simulink model "Telescope_model_PID"  (R2024b)
settings: Solver=ode4  StartTime=0.0  StopTime=SimulationTime  FixedStep=Tc  RelTol=1e-5
undefined symbols (not defined in the file): Arcs2Deg, Deg2Arcs, Kd_az, Kd_el, Ki_az, Ki_el, Kp_az, Kp_el, Kv, Prepocessor, Scenario, sgn, sysAz, sysEL, VonKarman
libraries: simulink x16
(part 1 of 2)
settings Model: Creator=giaco  LastModifiedBy=giacomobasile
settings RTWCC: GPUComputeCapability=3.5

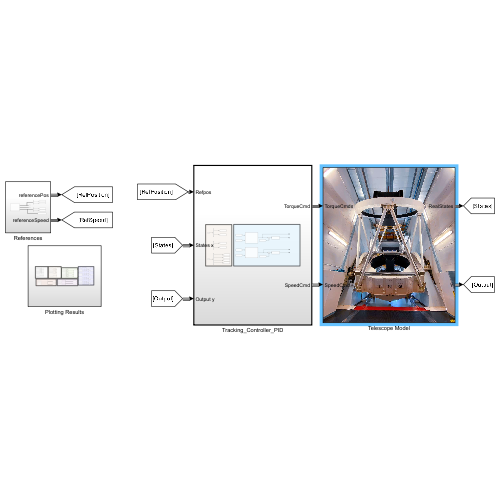
[thumbnail: Simulink's stored preview of the top-level diagram]
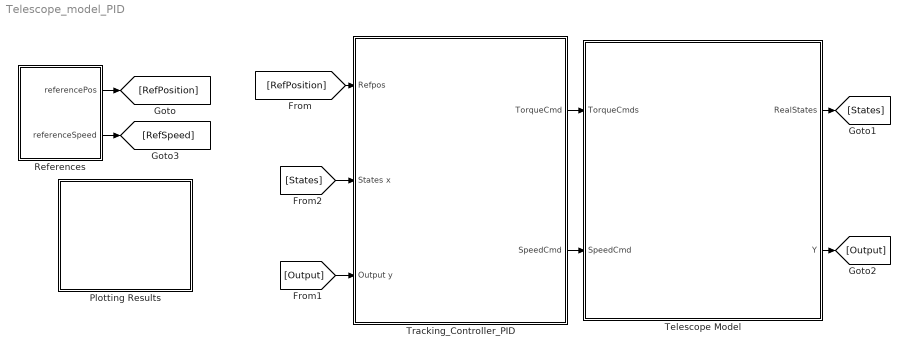
== system Telescope_model_PID ==
  Plotting Results : Subsystem
  References : Subsystem
  Telescope Model : Subsystem
      mask Display: image('tng1.jpg');
  Tracking_Controller_PID : Subsystem  TreatAsAtomicUnit=on  VariantControl=CtrMode == 1
  wires:
  Telescope Model/1(RealStates) -> [States]
  Telescope Model/2(Y) -> [Output]
  References/1(referencePos) -> [RefPosition]
  [RefPosition] -> Tracking_Controller_PID/1(Refpos)
  [States] -> Tracking_Controller_PID/2(States x)
  [Output] -> Tracking_Controller_PID/3(Output y)
  Tracking_Controller_PID/1(TorqueCmd) -> Telescope Model/1(TorqueCmds)
  Tracking_Controller_PID/2(SpeedCmd) -> Telescope Model/2(SpeedCmd)
  References/2(referenceSpeed) -> [RefSpeed]

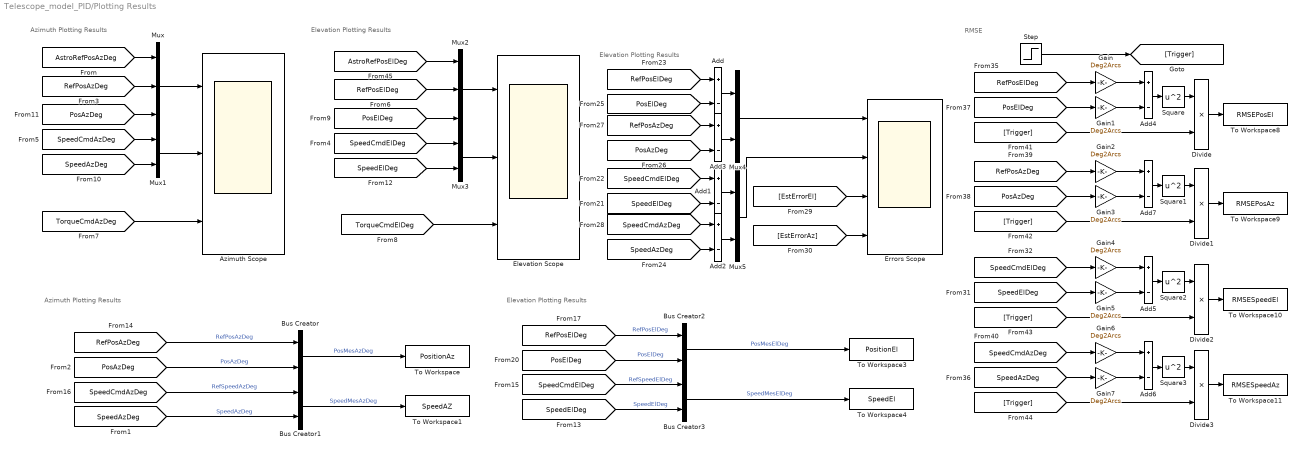
== system Telescope_model_PID/Plotting Results ==
  note: RMSE
  note: Azimuth Plotting Results
  note: Elevation Plotting Results
  note: Elevation Plotting Results
  note: Azimuth Plotting Results
  note: Elevation Plotting Results
  Add{,1..7} (8 alike) : Sum  Inputs=+-
  Azimuth Scope : Scope  NumInputPorts=3
  Bus Creator{,1..3} (4 alike) : BusCreator  Inputs=2
  Divide{,1..3} (4 alike) : Product  Inputs=**
  Elevation Scope : Scope  NumInputPorts=3
  Errors Scope : Scope  NumInputPorts=4
  Gain{,1..7} (8 alike) : Gain  Gain=Deg2Arcs
  Mux : Mux  Inputs=3
  Mux{1,3..5} (4 alike) : Mux  Inputs=2
  Mux2 : Mux  Inputs=3
  Square{,1..3} (4 alike) : Math  Operator=square
  Step : Step  Time=350  SampleTime=0
  To Workspace : ToWorkspace  VariableName=PositionAz  SaveFormat=Timeseries  SampleTime=-1
  To Workspace1 : ToWorkspace  VariableName=SpeedAZ  SaveFormat=Timeseries  SampleTime=-1
  To Workspace10 : ToWorkspace  VariableName=RMSESpeedEl  SaveFormat=Timeseries  SampleTime=-1
  To Workspace11 : ToWorkspace  VariableName=RMSESpeedAz  SaveFormat=Timeseries  SampleTime=-1
  To Workspace3 : ToWorkspace  VariableName=PositionEl  SaveFormat=Timeseries  SampleTime=-1
  To Workspace4 : ToWorkspace  VariableName=SpeedEl  SaveFormat=Timeseries  SampleTime=-1
  To Workspace8 : ToWorkspace  VariableName=RMSEPosEl  SaveFormat=Timeseries  SampleTime=-1
  To Workspace9 : ToWorkspace  VariableName=RMSEPosAz  SaveFormat=Timeseries  SampleTime=-1
  wires:
  [RefPosAzDeg] -> Mux/2
  [PosAzDeg] -> Mux/3
  [SpeedCmdAzDeg] -> Mux1/1
  [SpeedAzDeg] -> Mux1/2
  Mux/1 -> Azimuth Scope/1
  Mux1/1 -> Azimuth Scope/2
  [TorqueCmdAzDeg] -> Azimuth Scope/3
  [TorqueCmdElDeg] -> Elevation Scope/3
  Mux3/1 -> Elevation Scope/2
  Mux2/1 -> Elevation Scope/1
  [SpeedElDeg] -> Mux3/2
  [SpeedCmdElDeg] -> Mux3/1
  [PosElDeg] -> Mux2/3
  [RefPosElDeg] -> Mux2/2
  [PosAzDeg] -> Bus Creator/2  "PosAzDeg"
  [SpeedAzDeg] -> Bus Creator1/2  "SpeedAzDeg"
  [RefPosAzDeg] -> Bus Creator/1  "RefPosAzDeg"
  [SpeedCmdAzDeg] -> Bus Creator1/1  "RefSpeedAzDeg"
  [RefPosElDeg] -> Bus Creator2/1  "RefPosElDeg"
  [PosElDeg] -> Bus Creator2/2  "PosElDeg"
  [SpeedCmdElDeg] -> Bus Creator3/1  "RefSpeedElDeg"
  [SpeedElDeg] -> Bus Creator3/2  "SpeedElDeg"
  Bus Creator/1 -> To Workspace/1  "PosMesAzDeg"
  Bus Creator1/1 -> To Workspace1/1  "SpeedMesAzDeg"
  Bus Creator2/1 -> To Workspace3/1  "PosMesElDeg"
  Bus Creator3/1 -> To Workspace4/1  "SpeedMesElDeg"
  [RefPosElDeg] -> Add/1
  [PosElDeg] -> Add/2
  [SpeedCmdElDeg] -> Add1/1
  [SpeedElDeg] -> Add1/2
  [SpeedCmdAzDeg] -> Add2/1
  [SpeedAzDeg] -> Add2/2
  [RefPosAzDeg] -> Add3/1
  [PosAzDeg] -> Add3/2
  Add/1 -> Mux4/1
  Add3/1 -> Mux4/2
  Add1/1 -> Mux5/1
  Add2/1 -> Mux5/2
  Mux4/1 -> Errors Scope/1
  Mux5/1 -> Errors Scope/2
  [EstErrorEl] -> Errors Scope/3
  [EstErrorAz] -> Errors Scope/4
  Add6/1 -> Square3/1
  Add5/1 -> Square2/1
  Add7/1 -> Square1/1
  Add4/1 -> Square/1
  [PosAzDeg] -> Gain3/1
  [RefPosAzDeg] -> Gain2/1
  [SpeedAzDeg] -> Gain7/1
  [SpeedCmdAzDeg] -> Gain6/1
  [SpeedElDeg] -> Gain5/1
  [SpeedCmdElDeg] -> Gain4/1
  [PosElDeg] -> Gain1/1
  [RefPosElDeg] -> Gain/1
  Square/1 -> Divide/1
  Divide/1 -> To Workspace8/1
  Step/1 -> [Trigger]
  [Trigger] -> Divide/2
  [Trigger] -> Divide1/2
  Square1/1 -> Divide1/1
  Divide1/1 -> To Workspace9/1
  [Trigger] -> Divide2/2
  Square2/1 -> Divide2/1
  Divide2/1 -> To Workspace10/1
  [Trigger] -> Divide3/2
  Square3/1 -> Divide3/1
  Divide3/1 -> To Workspace11/1
  Gain/1 -> Add4/1
  Gain1/1 -> Add4/2
  Gain2/1 -> Add7/1
  Gain3/1 -> Add7/2
  Gain4/1 -> Add5/1
  Gain5/1 -> Add5/2
  Gain6/1 -> Add6/1
  Gain7/1 -> Add6/2
  [AstroRefPosElDeg] -> Mux2/1
  [AstroRefPosAzDeg] -> Mux/1

== system Telescope_model_PID/References ==
  Bus Selector : BusSelector  OutputSignals=Azimuth,Elevation
  Bus Selector1 : BusSelector  OutputSignals=ElevationPosition,AzimuthPosition
  References : Subsystem  Variant=on  VariantControl=Choice
  To Workspace : ToWorkspace  VariableName=AstroReference  SaveFormat=Timeseries  SampleTime=-1
  referencePos : Outport
  referenceSpeed : Outport  Port=2
  tag scope: AstroRefPosAzDeg=global, AstroRefPosElDeg=global, RefPosAzDeg=global, RefPosElDeg=global
  wires:
  References/1(referencePos) -> Bus Selector/1, referencePos/1  "[Arcs]"
  Bus Selector/1 -> [RefPosAzDeg]  "<Azimuth>"
  Bus Selector/2 -> [RefPosElDeg]  "<Elevation>"
  References/2(referenceSpeed) -> referenceSpeed/1  "[Arcs]"
  Bus Selector1/2 -> [AstroRefPosAzDeg]  "<AzimuthPosition>"
  Bus Selector1/1 -> [AstroRefPosElDeg]  "<ElevationPosition>"
  References/3(AstroReference) -> To Workspace/1, Bus Selector1/1  "[Arcs]"

== system Telescope_model_PID/Telescope Model ==
  note: Input Management Section
  note: Models dynamics
  TorqueCmds : Inport
  SpeedCmd : Inport  Port=2
  Azimuth Model 50 deg : Subsystem
  Bus Selector : BusSelector  OutputSignals=Elevation,Azimuth50
  Bus Selector1 : BusSelector  OutputSignals=Elevation,Azimuth50
  Elevation Model : Subsystem
  Integrator : Integrator  InitialCondition=Prepocessor.p0el*Deg2Arcs
  Integrator1 : Integrator  InitialCondition=Prepocessor.p0az*Deg2Arcs
  To Workspace1 : ToWorkspace  VariableName=TorqueAz  SaveFormat=Timeseries  SampleTime=-1
  To Workspace3 : ToWorkspace  VariableName=TorqueEl  SaveFormat=Timeseries  SampleTime=-1
  Transfer Fcn1 : TransferFcn  Numerator=10000  Denominator=conv([1 100], [1 100])
  Transfer Fcn2 : TransferFcn  Numerator=10000  Denominator=conv([1 100], [1 100])
  Out Bus Element : Outport  PortName=RealStates  Element=Elevation
  Out Bus Element1 : Outport  PortName=RealStates  Element=Azimuth50
  Out Bus Element2 : Outport  Port=2  PortName=Y  Element=ElevationSpeed
  Out Bus Element3 : Outport  Port=2  PortName=Y  Element=ElevationPosition
  Out Bus Element4 : Outport  Port=2  PortName=Y  Element=Azimuth50Speed
  Out Bus Element5 : Outport  Port=2  PortName=Y  Element=Azimuth50Position
  tag scope: PosAzDeg=global, PosElDeg=global, SpeedAzDeg=global, SpeedCmdAzDeg=global, SpeedCmdElDeg=global, SpeedElDeg=global, TorqueCmdAzDeg=global, TorqueCmdElDeg=global
  wires:
  Elevation Model/1(x) -> Out Bus Element/1
  Azimuth Model 50 deg/1(x) -> Out Bus Element1/1
  TorqueCmds/1 -> Bus Selector/1
  Azimuth Model 50 deg/2(y) -> [SpeedAzDeg], Out Bus Element4/1, Integrator1/1
  Elevation Model/2(y) -> [SpeedElDeg], Out Bus Element2/1, Integrator/1
  Integrator1/1 -> [PosAzDeg], Out Bus Element5/1
  Integrator/1 -> [PosElDeg], Out Bus Element3/1
  Bus Selector1/2 -> Transfer Fcn1/1  "<Azimuth50>"
  Bus Selector/1 -> To Workspace3/1, [TorqueCmdElDeg]  "<Elevation>"
  Bus Selector1/1 -> Transfer Fcn2/1  "<Elevation>"
  Bus Selector/2 -> To Workspace1/1, [TorqueCmdAzDeg]  "<Azimuth50>"
  [TorqueCmdElDeg] -> Elevation Model/1(Torque)
  [TorqueCmdAzDeg] -> Azimuth Model 50 deg/1(Troque)
  SpeedCmd/1 -> Bus Selector1/1
  Transfer Fcn2/1 -> [SpeedCmdElDeg]
  Transfer Fcn1/1 -> [SpeedCmdAzDeg]

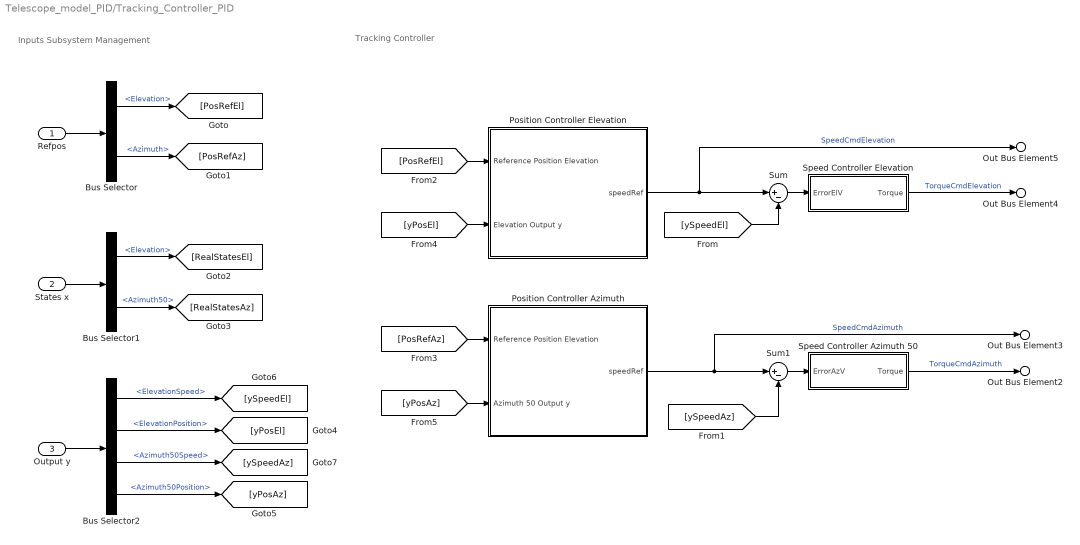
== system Telescope_model_PID/Tracking_Controller_PID ==
  note: Inputs Subsystem Management
  note: Tracking Controller
  Refpos : Inport
  States x : Inport  Port=2
  Output y : Inport  Port=3
  Bus Selector : BusSelector  OutputSignals=Elevation,Azimuth
  Bus Selector1 : BusSelector  OutputSignals=Elevation,Azimuth50
  Bus Selector2 : BusSelector  OutputSignals=ElevationSpeed,ElevationPosition,Azimuth50Speed,Azimuth50Position
  Position Controller Azimuth : Subsystem
  Position Controller Elevation : Subsystem
  Speed Controller Azimuth 50 : Subsystem
  Speed Controller Elevation : Subsystem
  Sum : Sum  Inputs=|+-
  Sum1 : Sum  Inputs=|+-
  Out Bus Element2 : Outport  PortName=TorqueCmd  Element=Azimuth50
  Out Bus Element4 : Outport  PortName=TorqueCmd  Element=Elevation
  Out Bus Element3 : Outport  Port=2  PortName=SpeedCmd  Element=Azimuth50
  Out Bus Element5 : Outport  Port=2  PortName=SpeedCmd  Element=Elevation
  wires:
  Position Controller Azimuth/1(speedRef) -> Sum1/1, Out Bus Element3/1  "SpeedCmdAzimuth"
  [PosRefEl] -> Position Controller Elevation/1(Reference Position Elevation)
  Sum/1 -> Speed Controller Elevation/1(ErrorElV)
  Sum1/1 -> Speed Controller Azimuth 50/1(ErrorAzV)
  [ySpeedAz] -> Sum1/2
  Speed Controller Azimuth 50/1(Torque) -> Out Bus Element2/1  "TorqueCmdAzimuth"
  Speed Controller Elevation/1(Torque) -> Out Bus Element4/1  "TorqueCmdElevation"
  Position Controller Elevation/1(speedRef) -> Sum/1, Out Bus Element5/1  "SpeedCmdElevation"
  [PosRefAz] -> Position Controller Azimuth/1(Reference Position Elevation)
  [ySpeedEl] -> Sum/2
  Bus Selector2/2 -> [yPosEl]  "<ElevationPosition>"
  Bus Selector2/1 -> [ySpeedEl]  "<ElevationSpeed>"
  Bus Selector2/3 -> [ySpeedAz]  "<Azimuth50Speed>"
  Bus Selector2/4 -> [yPosAz]  "<Azimuth50Position>"
  Output y/1 -> Bus Selector2/1
  Bus Selector1/2 -> [RealStatesAz]  "<Azimuth50>"
  Bus Selector1/1 -> [RealStatesEl]  "<Elevation>"
  States x/1 -> Bus Selector1/1
  Bus Selector/2 -> [PosRefAz]  "<Azimuth>"
  Bus Selector/1 -> [PosRefEl]  "<Elevation>"
  Refpos/1 -> Bus Selector/1
  [yPosEl] -> Position Controller Elevation/2(Elevation Output y)
  [yPosAz] -> Position Controller Azimuth/2(Azimuth 50 Output y)

== system Telescope_model_PID/References/References ==
  Astrometric Computation : Subsystem  VariantControl=Ref == 0 && Prepocessor.flag == 0 && TNG==0
  Constant Referemce : Subsystem  VariantControl=Ref == 2
  Preprocessed Astrometric Computation : Subsystem  VariantControl=Ref == 0 && Prepocessor.flag == 1 && TNG==0
  Preprocessed Astrometric References from TNG : Subsystem  VariantControl=Ref == 0 && Prepocessor.flag == 1 && TNG==1
  Trivial References PID/LQG : Subsystem  VariantControl=Ref == 1
  referencePos : Outport
  referenceSpeed : Outport  Port=2
  AstroReference : Outport  Port=3

== system Telescope_model_PID/Telescope Model/Azimuth Model 50 deg ==
  Troque : Inport
  Add : Sum
  Add1 : Sum
  Integrator : Integrator
  Noise Model : Subsystem  Variant=on  VariantControl=Choice
  Scope : Scope  NumInputPorts=2
  Sum : Sum  Inputs=++|
  Sum1 : Sum  Inputs=++|
  sys.A : Gain  Gain=sysAz.A  Multiplication=Matrix(K*u)
  sys.B : Gain  Gain=sysAz.B  Multiplication=Matrix(K*u)
  sys.C : Gain  Gain=sysAz.C  Multiplication=Matrix(K*u)
  sys.D : Gain  Gain=sysAz.D  Multiplication=Matrix(K*u)
  x : Outport
  y : Outport  Port=2
  tag scope: InputNoiseAz=global
  wires:
  Add1/1 -> Integrator/1
  sys.C/1 -> Add/2
  sys.D/1 -> Add/1
  Sum1/1 -> sys.B/1, sys.D/1
  Sum/1 -> y/1
  Add/1 -> Sum/2
  Troque/1 -> Sum1/2
  Noise Model/1(d_out) -> Scope/1, Sum/1
  sys.B/1 -> Add1/1
  sys.A/1 -> Add1/2
  Integrator/1 -> sys.A/1, sys.C/1, x/1
  Noise Model/2(d_in) -> [InputNoiseAz], Sum1/1, Scope/2

== system Telescope_model_PID/Telescope Model/Elevation Model ==
  Torque : Inport
  Add : Sum
  Add1 : Sum
  Integrator : Integrator
  Noise Model : Subsystem  Variant=on  VariantControl=Choice
  Scope : Scope  NumInputPorts=2
  Sum : Sum  Inputs=++|
  Sum1 : Sum  Inputs=++|
  sys.A : Gain  Gain=sysEL.A  Multiplication=Matrix(K*u)
  sys.B : Gain  Gain=sysEL.B  Multiplication=Matrix(K*u)
  sys.C : Gain  Gain=sysEL.C  Multiplication=Matrix(K*u)
  sys.D : Gain  Gain=sysEL.D  Multiplication=Matrix(K*u)
  x : Outport
  y : Outport  Port=2
  tag scope: InputNoiseEl=global
  wires:
  sys.B/1 -> Add1/1
  sys.C/1 -> Add/2
  sys.D/1 -> Add/1
  Add/1 -> Sum/2
  Sum/1 -> y/1
  Sum1/1 -> sys.B/1, sys.D/1
  Torque/1 -> Sum1/2
  Noise Model/1(d_out) -> Scope/1, Sum/1
  Noise Model/2(d_in) -> [InputNoiseEl], Sum1/1, Scope/2
  sys.A/1 -> Add1/2
  Add1/1 -> Integrator/1
  Integrator/1 -> sys.A/1, x/1, sys.C/1

== system Telescope_model_PID/Tracking_Controller_PID/Position Controller Azimuth ==
  note: Inputs Subsystem Management
  note: Controller PID
  Reference Position Elevation : Inport
  Azimuth 50 Output y : Inport  Port=2
  Add4 : Sum  Inputs=+++
  Gain1 : Gain  Gain=Kd_az  Multiplication=Matrix(K*u)
  Gain5 : Gain  Gain=Kp_az  Multiplication=Matrix(K*u)
  Gain6 : Gain  Gain=Ki_az  Multiplication=Matrix(K*u)
  Integrator : Integrator
  Sum : Sum  Inputs=+-|
  Transfer Fcn : TransferFcn  Numerator=[100 0]  Denominator=[1 100]
  speedRef : Outport
  wires:
  Reference Position Elevation/1 -> Sum/1
  Azimuth 50 Output y/1 -> Sum/2
  Sum/1 -> [ErrorP]
  Add4/1 -> speedRef/1
  Transfer Fcn/1 -> Gain1/1
  [ErrorP] -> Gain5/1, Transfer Fcn/1, Integrator/1
  Gain6/1 -> Add4/2
  Gain5/1 -> Add4/1
  Integrator/1 -> Gain6/1
  Gain1/1 -> Add4/3

== system Telescope_model_PID/Tracking_Controller_PID/Position Controller Elevation ==
  note: Inputs Subsystem Management
  note: Controller PID
  Reference Position Elevation : Inport
  Elevation Output y : Inport  Port=2
  Add4 : Sum  Inputs=+++
  Gain1 : Gain  Gain=Kd_el  Multiplication=Matrix(K*u)
  Gain5 : Gain  Gain=Kp_el  Multiplication=Matrix(K*u)
  Gain6 : Gain  Gain=Ki_el  Multiplication=Matrix(K*u)
  Integrator : Integrator
  Sum : Sum  Inputs=+-|
  Transfer Fcn : TransferFcn  Numerator=[100 0]  Denominator=[1 100]
  speedRef : Outport
  wires:
  Reference Position Elevation/1 -> Sum/1
  Gain6/1 -> Add4/2
  Integrator/1 -> Gain6/1
  [ErrorP] -> Gain5/1, Transfer Fcn/1, Integrator/1
  Gain5/1 -> Add4/1
  Sum/1 -> [ErrorP]
  Elevation Output y/1 -> Sum/2
  Add4/1 -> speedRef/1
  Transfer Fcn/1 -> Gain1/1
  Gain1/1 -> Add4/3

== system Telescope_model_PID/Tracking_Controller_PID/Speed Controller Azimuth 50 ==
  ErrorAzV : Inport
  Gain : Gain  Gain=Kv
  Integrator : Integrator
  Torque : Outport
  wires:
  Gain/1 -> Torque/1
  ErrorAzV/1 -> Integrator/1
  Integrator/1 -> Gain/1

== system Telescope_model_PID/Tracking_Controller_PID/Speed Controller Elevation ==
  ErrorElV : Inport
  Gain : Gain  Gain=-Kv
  Integrator : Integrator
  Torque : Outport
  wires:
  Integrator/1 -> Gain/1
  ErrorElV/1 -> Integrator/1
  Gain/1 -> Torque/1

== system Telescope_model_PID/References/References/Astrometric Computation ==
  Clock : Clock
  Constant10 : Constant  Value=Scenario.VLT
  Constant11 : Constant  Value=Scenario.Time
  Constant19 : Constant  Value=Scenario.RAhh
  Constant21 : Constant  Value=Scenario.DECdd
  Constant3 : Constant  Value=Scenario.RAmm
  Constant4 : Constant  Value=Scenario.RAss
  Constant6 : Constant  Value=Scenario.DECmm
  Constant7 : Constant  Value=Scenario.DECss
  Constant8 : Constant  Value=Scenario.LATsite
  Constant9 : Constant  Value=Scenario.LONsite
  Discrete Derivative{,1..3} (4 alike) : simulink/Discrete/Discrete Derivative  gainval=1.0  ICPrevScaledInput=0.0  OutMin=[]  OutMax=[]  OutDataType=fixdt(1, 16)  OutScaling=2^-10  DoSatur=off
  MATLAB Function : MATLAB Function  TreatAsAtomicUnit=on
  Scope2 : Scope
  Out Bus Element : Outport  PortName=referencePos  Element=Azimuth
  Out Bus Element1 : Outport  PortName=referencePos  Element=Elevation
  Out Bus Element2 : Outport  Port=2  PortName=referenceSpeed  Element=Azimuth
  Out Bus Element3 : Outport  Port=2  PortName=referenceSpeed  Element=Elevation
  Out Bus Element4 : Outport  Port=3  PortName=AstroReference  Element=AzimuthSpeed
  Out Bus Element5 : Outport  Port=3  PortName=AstroReference  Element=ElevationPosition
  Out Bus Element6 : Outport  Port=3  PortName=AstroReference  Element=AzimuthPosition
  Out Bus Element7 : Outport  Port=3  PortName=AstroReference  Element=ElevationSpeed
  wires:
  Discrete Derivative1/1 -> Out Bus Element7/1
  Constant9/1 -> MATLAB Function/10(Longitude)
  Constant19/1 -> MATLAB Function/3(RAhh)
  Constant3/1 -> MATLAB Function/4(RAmm)
  Constant21/1 -> MATLAB Function/6(DECdd)
  Clock/1 -> Scope2/1, MATLAB Function/1(clo)
  Discrete Derivative3/1 -> Out Bus Element3/1
  Constant4/1 -> MATLAB Function/5(RAss)
  Constant7/1 -> MATLAB Function/8(DECss)
  Constant6/1 -> MATLAB Function/7(DECmm)
  Constant10/1 -> MATLAB Function/11(VLT)
  Constant11/1 -> MATLAB Function/2(Time)
  Discrete Derivative2/1 -> Out Bus Element2/1
  Constant8/1 -> MATLAB Function/9(Latitude)
  MATLAB Function/1(Az) -> Discrete Derivative/1, Out Bus Element6/1, Discrete Derivative2/1, Out Bus Element/1
  MATLAB Function/2(Alt) -> Discrete Derivative3/1, Out Bus Element5/1, Discrete Derivative1/1, Out Bus Element1/1
  Discrete Derivative/1 -> Out Bus Element4/1

== system Telescope_model_PID/References/References/Constant Referemce ==
  Constant2 : Constant  Value=0
  Constant3 : Constant  Value=0
  Discrete Derivative : simulink/Discrete/Discrete Derivative  gainval=1.0  ICPrevScaledInput=0.0  OutMin=[]  OutMax=[]  OutDataType=fixdt(1, 16)  OutScaling=2^-10  DoSatur=off
  Discrete Derivative1 : simulink/Discrete/Discrete Derivative  gainval=1.0  ICPrevScaledInput=0.0  OutMin=[]  OutMax=[]  OutDataType=fixdt(1, 16)  OutScaling=2^-10  DoSatur=off
  Gain{6..13} (8 alike) : Gain  Gain=Deg2Arcs
  Integrator3 : Integrator  InitialCondition=120
  Integrator4 : Integrator  InitialCondition=60
  Prepocessor Azimuth : Subsystem
  Prepocessor Elavation : Subsystem
  Out Bus Element : Outport  PortName=referencePos  Element=Azimuth
  Out Bus Element1 : Outport  PortName=referencePos  Element=Elevation
  Out Bus Element2 : Outport  Port=2  PortName=referenceSpeed  Element=Azimuth
  Out Bus Element3 : Outport  Port=2  PortName=referenceSpeed  Element=Elevation
  Out Bus Element4 : Outport  Port=3  PortName=AstroReference  Element=AzimuthSpeed
  Out Bus Element5 : Outport  Port=3  PortName=AstroReference  Element=ElevationPosition
  Out Bus Element6 : Outport  Port=3  PortName=AstroReference  Element=AzimuthPosition
  Out Bus Element7 : Outport  Port=3  PortName=AstroReference  Element=ElevationSpeed
  wires:
  Integrator3/1 -> Discrete Derivative1/1, Gain8/1, Prepocessor Azimuth/1(Astrometry Computation)  "[Deg]"
  Integrator4/1 -> Prepocessor Elavation/1(Astrometry Computation), Discrete Derivative/1, Gain11/1  "[Deg]"
  Prepocessor Elavation/1(ReferencePosition) -> Gain12/1
  Prepocessor Azimuth/1(ReferencePosition) -> Gain6/1
  Gain8/1 -> Out Bus Element6/1
  Gain10/1 -> Out Bus Element7/1
  Gain11/1 -> Out Bus Element5/1
  Gain6/1 -> Out Bus Element/1
  Gain13/1 -> Out Bus Element3/1
  Gain7/1 -> Out Bus Element2/1
  Discrete Derivative1/1 -> Gain9/1
  Discrete Derivative/1 -> Gain10/1
  Gain12/1 -> Out Bus Element1/1
  Prepocessor Elavation/2(ReferenceSpeed) -> Gain13/1
  Constant3/1 -> Integrator4/1  "[Deg]"
  Gain9/1 -> Out Bus Element4/1
  Constant2/1 -> Integrator3/1  "[Deg]"
  Prepocessor Azimuth/2(ReferenceSpeed) -> Gain7/1

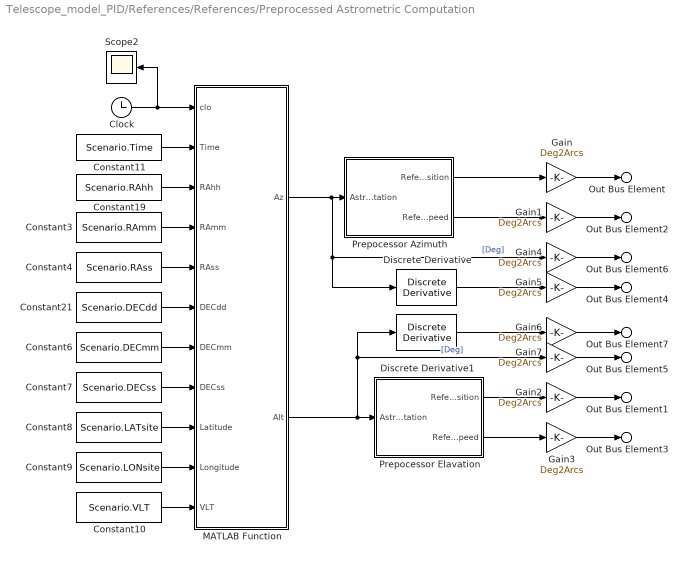
== system Telescope_model_PID/References/References/Preprocessed Astrometric Computation ==
  Clock : Clock
  Constant10 : Constant  Value=Scenario.VLT
  Constant11 : Constant  Value=Scenario.Time
  Constant19 : Constant  Value=Scenario.RAhh
  Constant21 : Constant  Value=Scenario.DECdd
  Constant3 : Constant  Value=Scenario.RAmm
  Constant4 : Constant  Value=Scenario.RAss
  Constant6 : Constant  Value=Scenario.DECmm
  Constant7 : Constant  Value=Scenario.DECss
  Constant8 : Constant  Value=Scenario.LATsite
  Constant9 : Constant  Value=Scenario.LONsite
  Discrete Derivative : simulink/Discrete/Discrete Derivative  gainval=1.0  ICPrevScaledInput=0.0  OutMin=[]  OutMax=[]  OutDataType=fixdt(1, 16)  OutScaling=2^-10  DoSatur=off
  Discrete Derivative1 : simulink/Discrete/Discrete Derivative  gainval=1.0  ICPrevScaledInput=0.0  OutMin=[]  OutMax=[]  OutDataType=fixdt(1, 16)  OutScaling=2^-10  DoSatur=off
  Gain{,1..7} (8 alike) : Gain  Gain=Deg2Arcs
  MATLAB Function : MATLAB Function  TreatAsAtomicUnit=on
  Prepocessor Azimuth : Subsystem
  Prepocessor Elavation : Subsystem
  Scope2 : Scope
  Out Bus Element : Outport  PortName=referencePos  Element=Azimuth
  Out Bus Element1 : Outport  PortName=referencePos  Element=Elevation
  Out Bus Element2 : Outport  Port=2  PortName=referenceSpeed  Element=Azimuth
  Out Bus Element3 : Outport  Port=2  PortName=referenceSpeed  Element=Elevation
  Out Bus Element4 : Outport  Port=3  PortName=AstroReference  Element=AzimuthSpeed
  Out Bus Element5 : Outport  Port=3  PortName=AstroReference  Element=ElevationPosition
  Out Bus Element6 : Outport  Port=3  PortName=AstroReference  Element=AzimuthPosition
  Out Bus Element7 : Outport  Port=3  PortName=AstroReference  Element=ElevationSpeed
  wires:
  Constant21/1 -> MATLAB Function/6(DECdd)
  Constant7/1 -> MATLAB Function/8(DECss)
  Constant11/1 -> MATLAB Function/2(Time)
  Constant6/1 -> MATLAB Function/7(DECmm)
  Constant10/1 -> MATLAB Function/11(VLT)
  Clock/1 -> Scope2/1, MATLAB Function/1(clo)
  Constant4/1 -> MATLAB Function/5(RAss)
  Constant8/1 -> MATLAB Function/9(Latitude)
  Constant3/1 -> MATLAB Function/4(RAmm)
  Constant9/1 -> MATLAB Function/10(Longitude)
  Constant19/1 -> MATLAB Function/3(RAhh)
  MATLAB Function/1(Az) -> Gain4/1, Discrete Derivative/1, Prepocessor Azimuth/1(Astrometry Computation)  "[Deg]"
  MATLAB Function/2(Alt) -> Discrete Derivative1/1, Gain7/1, Prepocessor Elavation/1(Astrometry Computation)  "[Deg]"
  Prepocessor Azimuth/2(ReferenceSpeed) -> Gain1/1
  Prepocessor Azimuth/1(ReferencePosition) -> Gain/1
  Prepocessor Elavation/2(ReferenceSpeed) -> Gain3/1
  Prepocessor Elavation/1(ReferencePosition) -> Gain2/1
  Discrete Derivative/1 -> Gain5/1
  Discrete Derivative1/1 -> Gain6/1
  Gain/1 -> Out Bus Element/1
  Gain1/1 -> Out Bus Element2/1
  Gain2/1 -> Out Bus Element1/1
  Gain3/1 -> Out Bus Element3/1
  Gain4/1 -> Out Bus Element6/1
  Gain5/1 -> Out Bus Element4/1
  Gain6/1 -> Out Bus Element7/1
  Gain7/1 -> Out Bus Element5/1

== system Telescope_model_PID/References/References/Preprocessed Astrometric References from TNG ==
  Discrete Derivative : simulink/Discrete/Discrete Derivative  gainval=1.0  ICPrevScaledInput=0.0  OutMin=[]  OutMax=[]  OutDataType=fixdt(1, 16)  OutScaling=2^-10  DoSatur=off
  Discrete Derivative1 : simulink/Discrete/Discrete Derivative  gainval=1.0  ICPrevScaledInput=0.0  OutMin=[]  OutMax=[]  OutDataType=fixdt(1, 16)  OutScaling=2^-10  DoSatur=off
  From Workspace : FromWorkspace  VariableName=Scenario.AzimuthPosition
  From Workspace1 : FromWorkspace  VariableName=Scenario.ElevationPosition
  Gain : Gain  Gain=Arcs2Deg
  Gain1 : Gain  Gain=Arcs2Deg
  Gain{2..9} (8 alike) : Gain  Gain=Deg2Arcs
  Prepocessor Azimuth : Subsystem
  Prepocessor Elavation : Subsystem
  Out Bus Element : Outport  PortName=referencePos  Element=Azimuth
  Out Bus Element1 : Outport  PortName=referencePos  Element=Elevation
  Out Bus Element2 : Outport  Port=2  PortName=referenceSpeed  Element=Azimuth
  Out Bus Element3 : Outport  Port=2  PortName=referenceSpeed  Element=Elevation
  Out Bus Element4 : Outport  Port=3  PortName=AstroReference  Element=AzimuthSpeed
  Out Bus Element5 : Outport  Port=3  PortName=AstroReference  Element=ElevationPosition
  Out Bus Element6 : Outport  Port=3  PortName=AstroReference  Element=AzimuthPosition
  Out Bus Element7 : Outport  Port=3  PortName=AstroReference  Element=ElevationSpeed
  wires:
  Discrete Derivative/1 -> Gain6/1
  Discrete Derivative1/1 -> Gain5/1
  Prepocessor Elavation/1(ReferencePosition) -> Gain8/1
  Prepocessor Elavation/2(ReferenceSpeed) -> Gain9/1
  Prepocessor Azimuth/1(ReferencePosition) -> Gain2/1
  Prepocessor Azimuth/2(ReferenceSpeed) -> Gain3/1
  From Workspace/1 -> Gain/1  "[Arcs]"
  Gain/1 -> Prepocessor Azimuth/1(Astrometry Computation), Discrete Derivative1/1, Gain4/1  "[Deg]"
  Gain1/1 -> Prepocessor Elavation/1(Astrometry Computation), Discrete Derivative/1, Gain7/1  "[Deg]"
  From Workspace1/1 -> Gain1/1  "[Arcs]"
  Gain2/1 -> Out Bus Element/1
  Gain3/1 -> Out Bus Element2/1
  Gain4/1 -> Out Bus Element6/1
  Gain5/1 -> Out Bus Element4/1
  Gain6/1 -> Out Bus Element7/1
  Gain7/1 -> Out Bus Element5/1
  Gain8/1 -> Out Bus Element1/1
  Gain9/1 -> Out Bus Element3/1

== system Telescope_model_PID/References/References/Trivial References PID//LQG ==
  Add1 : Sum  Inputs=+-
  Add2 : Sum  Inputs=+-
  Discrete Derivative : simulink/Discrete/Discrete Derivative  gainval=1.0  ICPrevScaledInput=0.0  OutMin=[]  OutMax=[]  OutDataType=fixdt(1, 16)  OutScaling=2^-10  DoSatur=off
  Discrete Derivative1 : simulink/Discrete/Discrete Derivative  gainval=1.0  ICPrevScaledInput=0.0  OutMin=[]  OutMax=[]  OutDataType=fixdt(1, 16)  OutScaling=2^-10  DoSatur=off
  Gain{6..13} (8 alike) : Gain  Gain=Deg2Arcs
  Integrator1 : Integrator
  Integrator2 : Integrator
  Prepocessor Azimuth : Subsystem
  Prepocessor Elavation : Subsystem
  Step1 : Step  Time=2  After=5  SampleTime=0
  Step2 : Step  Time=12  After=5  SampleTime=0
  Step4 : Step  Time=20  After=0.2  SampleTime=0
  Step5 : Step  Time=30  After=0.2  SampleTime=0
  Out Bus Element : Outport  PortName=referencePos  Element=Azimuth
  Out Bus Element1 : Outport  PortName=referencePos  Element=Elevation
  Out Bus Element2 : Outport  Port=2  PortName=referenceSpeed  Element=Azimuth
  Out Bus Element3 : Outport  Port=2  PortName=referenceSpeed  Element=Elevation
  Out Bus Element4 : Outport  Port=3  PortName=AstroReference  Element=AzimuthSpeed
  Out Bus Element5 : Outport  Port=3  PortName=AstroReference  Element=ElevationPosition
  Out Bus Element6 : Outport  Port=3  PortName=AstroReference  Element=AzimuthPosition
  Out Bus Element7 : Outport  Port=3  PortName=AstroReference  Element=ElevationSpeed
  wires:
  Step4/1 -> Add2/1
  Step5/1 -> Add2/2
  Step2/1 -> Add1/2
  Step1/1 -> Add1/1
  Add1/1 -> Integrator1/1  "[Deg]"
  Add2/1 -> Integrator2/1  "[Deg]"
  Gain6/1 -> Out Bus Element/1
  Gain11/1 -> Out Bus Element5/1
  Gain10/1 -> Out Bus Element7/1
  Gain7/1 -> Out Bus Element2/1
  Gain13/1 -> Out Bus Element3/1
  Gain9/1 -> Out Bus Element4/1
  Prepocessor Azimuth/2(ReferenceSpeed) -> Gain7/1
  Prepocessor Azimuth/1(ReferencePosition) -> Gain6/1
  Prepocessor Elavation/1(ReferencePosition) -> Gain12/1
  Prepocessor Elavation/2(ReferenceSpeed) -> Gain13/1
  Gain8/1 -> Out Bus Element6/1
  Integrator1/1 -> Discrete Derivative1/1, Gain8/1, Prepocessor Azimuth/1(Astrometry Computation)  "[Deg]"
  Integrator2/1 -> Prepocessor Elavation/1(Astrometry Computation), Discrete Derivative/1, Gain11/1  "[Deg]"
  Gain12/1 -> Out Bus Element1/1
  Discrete Derivative1/1 -> Gain9/1
  Discrete Derivative/1 -> Gain10/1

== system Telescope_model_PID/Telescope Model/Azimuth Model 50 deg/Noise Model ==
  None Noise : Subsystem  VariantControl="NNFConf  == 0"
  Von Karman Torque PSD : Subsystem  VariantControl=NNFConf == 2
  White Noise Output : Subsystem  VariantControl=NNFConf == 1
  d_out : Outport
  d_in : Outport  Port=2

== system Telescope_model_PID/Telescope Model/Elevation Model/Noise Model ==
  None Noise : Subsystem  VariantControl="NNFConf  == 0"
  Von Karman Torque PSD : Subsystem  VariantControl=NNFConf == 2
  White Noise Output : Subsystem  VariantControl=NNFConf == 1
  d_out : Outport
  d_in : Outport  Port=2

== system Telescope_model_PID/References/References/Constant Referemce/Prepocessor Azimuth ==
  Astrometry Computation : Inport
  Integrator : Integrator  InitialCondition=Prepocessor.p0az
  Prepocessor Elevation : Subsystem  TreatAsAtomicUnit=on  SystemSampleTime=Prepocessor.Ts
  Terminator : Terminator
  Terminator1 : Terminator
  To Workspace : ToWorkspace  VariableName=ReferenceProcessedPositionAz  SaveFormat=Timeseries  SampleTime=-1
  To Workspace1 : ToWorkspace  VariableName=ReferenceProcessedSpeedAz  SaveFormat=Timeseries  SampleTime=-1
  Transfer Fcn2 : TransferFcn  Numerator=2500  Denominator=conv([1 50], [1 50])
  ReferencePosition : Outport
  ReferenceSpeed : Outport  Port=2
  wires:
  Prepocessor Elevation/2(speed) -> Transfer Fcn2/1
  Prepocessor Elevation/1(deltaP) -> Terminator/1
  Integrator/1 -> To Workspace/1, ReferencePosition/1
  Prepocessor Elevation/3(PositionRef) -> Terminator1/1
  Transfer Fcn2/1 -> To Workspace1/1, ReferenceSpeed/1, Integrator/1
  Astrometry Computation/1 -> Prepocessor Elevation/1(Az)

== system Telescope_model_PID/References/References/Constant Referemce/Prepocessor Elavation ==
  Astrometry Computation : Inport
  Integrator : Integrator  InitialCondition=Prepocessor.p0el
  Prepocessor Elevation : Subsystem  TreatAsAtomicUnit=on  SystemSampleTime=Prepocessor.Ts
  Terminator : Terminator
  Terminator1 : Terminator
  To Workspace : ToWorkspace  VariableName=ReferenceProcessedPositionEl  SaveFormat=Timeseries  SampleTime=-1
  To Workspace1 : ToWorkspace  VariableName=ReferenceProcessedSpeedEl  SaveFormat=Timeseries  SampleTime=-1
  Transfer Fcn2 : TransferFcn  Numerator=2500  Denominator=conv([1 50], [1 50])
  ReferencePosition : Outport
  ReferenceSpeed : Outport  Port=2
  wires:
  Transfer Fcn2/1 -> Integrator/1, To Workspace1/1, ReferenceSpeed/1
  Prepocessor Elevation/3(PositionRef) -> Terminator1/1
  Integrator/1 -> To Workspace/1, ReferencePosition/1
  Prepocessor Elevation/1(deltaP) -> Terminator/1
  Prepocessor Elevation/2(speed) -> Transfer Fcn2/1
  Astrometry Computation/1 -> Prepocessor Elevation/1(El)

== system Telescope_model_PID/References/References/Preprocessed Astrometric Computation/Prepocessor Azimuth ==
  Astrometry Computation : Inport
  Integrator : Integrator  InitialCondition=Prepocessor.p0az
  Prepocessor Elevation : Subsystem  TreatAsAtomicUnit=on  SystemSampleTime=Prepocessor.Ts
  Terminator : Terminator
  Terminator1 : Terminator
  To Workspace : ToWorkspace  VariableName=ReferenceProcessedPositionAz  SaveFormat=Timeseries  SampleTime=-1
  To Workspace1 : ToWorkspace  VariableName=ReferenceProcessedSpeedAz  SaveFormat=Timeseries  SampleTime=-1
  Transfer Fcn2 : TransferFcn  Numerator=2500  Denominator=conv([1 50], [1 50])
  ReferencePosition : Outport
  ReferenceSpeed : Outport  Port=2
  wires:
  Prepocessor Elevation/2(speed) -> Transfer Fcn2/1
  Prepocessor Elevation/1(deltaP) -> Terminator/1
  Integrator/1 -> To Workspace/1, ReferencePosition/1
  Prepocessor Elevation/3(PositionRef) -> Terminator1/1
  Transfer Fcn2/1 -> To Workspace1/1, ReferenceSpeed/1, Integrator/1
  Astrometry Computation/1 -> Prepocessor Elevation/1(Az)

== system Telescope_model_PID/References/References/Preprocessed Astrometric Computation/Prepocessor Elavation ==
  Astrometry Computation : Inport
  Integrator : Integrator  InitialCondition=Prepocessor.p0el
  Prepocessor Elevation : Subsystem  TreatAsAtomicUnit=on  SystemSampleTime=Prepocessor.Ts
  Terminator : Terminator
  Terminator1 : Terminator
  To Workspace : ToWorkspace  VariableName=ReferenceProcessedPositionEl  SaveFormat=Timeseries  SampleTime=-1
  To Workspace1 : ToWorkspace  VariableName=ReferenceProcessedSpeedEl  SaveFormat=Timeseries  SampleTime=-1
  Transfer Fcn2 : TransferFcn  Numerator=2500  Denominator=conv([1 50], [1 50])
  ReferencePosition : Outport
  ReferenceSpeed : Outport  Port=2
  wires:
  Transfer Fcn2/1 -> Integrator/1, To Workspace1/1, ReferenceSpeed/1
  Prepocessor Elevation/3(PositionRef) -> Terminator1/1
  Integrator/1 -> To Workspace/1, ReferencePosition/1
  Prepocessor Elevation/1(deltaP) -> Terminator/1
  Prepocessor Elevation/2(speed) -> Transfer Fcn2/1
  Astrometry Computation/1 -> Prepocessor Elevation/1(El)

== system Telescope_model_PID/References/References/Preprocessed Astrometric References from TNG/Prepocessor Azimuth ==
  Astrometry Computation : Inport
  Integrator : Integrator  InitialCondition=Prepocessor.p0az
  Prepocessor Elevation : Subsystem  TreatAsAtomicUnit=on  SystemSampleTime=Prepocessor.Ts
  Terminator : Terminator
  Terminator1 : Terminator
  To Workspace : ToWorkspace  VariableName=ReferenceProcessedPositionAz  SaveFormat=Timeseries  SampleTime=-1
  To Workspace1 : ToWorkspace  VariableName=ReferenceProcessedSpeedAz  SaveFormat=Timeseries  SampleTime=-1
  Transfer Fcn2 : TransferFcn  Numerator=2500  Denominator=conv([1 50], [1 50])
  ReferencePosition : Outport
  ReferenceSpeed : Outport  Port=2
  wires:
  Prepocessor Elevation/2(speed) -> Transfer Fcn2/1
  Prepocessor Elevation/1(deltaP) -> Terminator/1
  Integrator/1 -> To Workspace/1, ReferencePosition/1
  Prepocessor Elevation/3(PositionRef) -> Terminator1/1
  Transfer Fcn2/1 -> To Workspace1/1, ReferenceSpeed/1, Integrator/1
  Astrometry Computation/1 -> Prepocessor Elevation/1(Az)

== system Telescope_model_PID/References/References/Preprocessed Astrometric References from TNG/Prepocessor Elavation ==
  Astrometry Computation : Inport
  Integrator : Integrator  InitialCondition=Prepocessor.p0el
  Prepocessor Elevation : Subsystem  TreatAsAtomicUnit=on  SystemSampleTime=Prepocessor.Ts
  Terminator : Terminator
  Terminator1 : Terminator
  To Workspace : ToWorkspace  VariableName=ReferenceProcessedPositionEl  SaveFormat=Timeseries  SampleTime=-1
  To Workspace1 : ToWorkspace  VariableName=ReferenceProcessedSpeedEl  SaveFormat=Timeseries  SampleTime=-1
  Transfer Fcn2 : TransferFcn  Numerator=2500  Denominator=conv([1 50], [1 50])
  ReferencePosition : Outport
  ReferenceSpeed : Outport  Port=2
  wires:
  Transfer Fcn2/1 -> Integrator/1, To Workspace1/1, ReferenceSpeed/1
  Prepocessor Elevation/3(PositionRef) -> Terminator1/1
  Integrator/1 -> To Workspace/1, ReferencePosition/1
  Prepocessor Elevation/1(deltaP) -> Terminator/1
  Prepocessor Elevation/2(speed) -> Transfer Fcn2/1
  Astrometry Computation/1 -> Prepocessor Elevation/1(El)

== system Telescope_model_PID/References/References/Trivial References PID//LQG/Prepocessor Azimuth ==
  Astrometry Computation : Inport
  Integrator : Integrator  InitialCondition=Prepocessor.p0az
  Prepocessor Elevation : Subsystem  TreatAsAtomicUnit=on  SystemSampleTime=Prepocessor.Ts
  Terminator : Terminator
  Terminator1 : Terminator
  To Workspace : ToWorkspace  VariableName=ReferenceProcessedPositionAz  SaveFormat=Timeseries  SampleTime=-1
  To Workspace1 : ToWorkspace  VariableName=ReferenceProcessedSpeedAz  SaveFormat=Timeseries  SampleTime=-1
  Transfer Fcn2 : TransferFcn  Numerator=2500  Denominator=conv([1 50], [1 50])
  ReferencePosition : Outport
  ReferenceSpeed : Outport  Port=2
  wires:
  Prepocessor Elevation/2(speed) -> Transfer Fcn2/1
  Prepocessor Elevation/1(deltaP) -> Terminator/1
  Integrator/1 -> To Workspace/1, ReferencePosition/1
  Prepocessor Elevation/3(PositionRef) -> Terminator1/1
  Transfer Fcn2/1 -> To Workspace1/1, ReferenceSpeed/1, Integrator/1
  Astrometry Computation/1 -> Prepocessor Elevation/1(Az)

== system Telescope_model_PID/References/References/Trivial References PID//LQG/Prepocessor Elavation ==
  Astrometry Computation : Inport
  Integrator : Integrator  InitialCondition=Prepocessor.p0el
  Prepocessor Elevation : Subsystem  TreatAsAtomicUnit=on  SystemSampleTime=Prepocessor.Ts
  Terminator : Terminator
  Terminator1 : Terminator
  To Workspace : ToWorkspace  VariableName=ReferenceProcessedPositionEl  SaveFormat=Timeseries  SampleTime=-1
  To Workspace1 : ToWorkspace  VariableName=ReferenceProcessedSpeedEl  SaveFormat=Timeseries  SampleTime=-1
  Transfer Fcn2 : TransferFcn  Numerator=2500  Denominator=conv([1 50], [1 50])
  ReferencePosition : Outport
  ReferenceSpeed : Outport  Port=2
  wires:
  Transfer Fcn2/1 -> Integrator/1, To Workspace1/1, ReferenceSpeed/1
  Prepocessor Elevation/3(PositionRef) -> Terminator1/1
  Integrator/1 -> To Workspace/1, ReferencePosition/1
  Prepocessor Elevation/1(deltaP) -> Terminator/1
  Prepocessor Elevation/2(speed) -> Transfer Fcn2/1
  Astrometry Computation/1 -> Prepocessor Elevation/1(El)

== system Telescope_model_PID/Telescope Model/Azimuth Model 50 deg/Noise Model/None Noise ==
  Clock : Clock
  Constant : Constant  Value=0
  Constant3 : Constant  Value=0
  Divide : Product  Inputs=**
  Divide1 : Product  Inputs=**
  d_out : Outport
  d_in : Outport  Port=2
  wires:
  Constant3/1 -> Divide/2
  Constant/1 -> Divide1/1
  Clock/1 -> Divide/1, Divide1/2
  Divide1/1 -> d_out/1
  Divide/1 -> d_in/1

== system Telescope_model_PID/Telescope Model/Azimuth Model 50 deg/Noise Model/Von Karman Torque PSD ==
  Add : Sum  Inputs=+
  Add2 : Sum
  Clock2 : Clock
  Constant : Constant  Value=0
  Constant1 : Constant  Value=4/VonKarman.v_mean^2
  Constant2 : Constant  Value=100
  Constant3 : Constant  Value=VonKarman.f
  Constant4 : Constant  Value=VonKarman.phi
  Cos1 : Trigonometry  Operator=cos
  Divide{1..6} (6 alike) : Product  Inputs=**
  Gain : Gain  Gain=VonKarman.alpha
  Gain1 : Gain  Gain=2*VonKarman.df
  Gain2 : Gain  Gain=2*pi
  Sqrt : Sqrt
  Square : Math  Operator=square
  Square1 : Math  Operator=square
  Step : Step  SampleTime=0
  Sv : Subsystem
  Transfer Fcn : TransferFcn  Numerator=[100]  Denominator=conv([1 10], [1 10])
  X : Subsystem
  d_out : Outport
  d_in : Outport  Port=2
  wires:
  Divide1/1 -> Transfer Fcn/1
  Cos1/1 -> Divide3/1
  Step/1 -> Divide1/2
  Divide4/1 -> Add2/1
  Gain1/1 -> Sqrt/1
  X/1(Out_X) -> Square/1
  Sqrt/1 -> Divide5/1
  Gain2/1 -> Divide4/2
  Clock2/1 -> Divide4/1
  Sv/1(Out_Sv) -> Divide2/2
  Constant2/1 -> Square1/1
  Add2/1 -> Cos1/1
  Divide2/1 -> Gain1/1
  Divide3/1 -> Add/1
  Square/1 -> Divide2/1
  Add/1 -> Divide1/1
  Constant1/1 -> Divide6/1
  Constant3/1 -> X/1(f), Sv/1(f), Gain2/1
  Divide5/1 -> Divide3/2
  Constant4/1 -> Add2/2
  Square1/1 -> Divide6/2
  Divide6/1 -> Divide5/2
  Transfer Fcn/1 -> Gain/1
  Constant/1 -> d_out/1
  Gain/1 -> d_in/1

== system Telescope_model_PID/Telescope Model/Azimuth Model 50 deg/Noise Model/White Noise Output ==
  Band-Limited White Noise : simulink/Sources/Band-Limited White Noise  Cov=[0.04]  Ts=0.02  seed=[23341]
  Band-Limited White Noise1 : simulink/Sources/Band-Limited White Noise  Cov=400000  Ts=0.02  seed=[23341]
  Constant1 : Constant  Value=0
  Gain : Gain  Gain=Deg2Arcs
  Scope : Scope  NumInputPorts=3
  d_out : Outport
  d_in : Outport  Port=2
  wires:
  Band-Limited White Noise/1 -> Scope/1, Gain/1
  Band-Limited White Noise1/1 -> Scope/2
  Gain/1 -> Scope/3, d_out/1
  Constant1/1 -> d_in/1

== system Telescope_model_PID/Telescope Model/Elevation Model/Noise Model/None Noise ==
  Clock : Clock
  Constant : Constant  Value=0
  Constant3 : Constant  Value=0
  Divide : Product  Inputs=**
  Divide1 : Product  Inputs=**
  d_out : Outport
  d_in : Outport  Port=2
  wires:
  Constant3/1 -> Divide/2
  Constant/1 -> Divide1/1
  Clock/1 -> Divide/1, Divide1/2
  Divide1/1 -> d_out/1
  Divide/1 -> d_in/1

== system Telescope_model_PID/Telescope Model/Elevation Model/Noise Model/Von Karman Torque PSD ==
  Add : Sum  Inputs=+
  Add2 : Sum
  Clock2 : Clock
  Constant : Constant  Value=0
  Constant1 : Constant  Value=4/VonKarman.v_mean^2
  Constant2 : Constant  Value=100
  Constant3 : Constant  Value=VonKarman.f
  Constant4 : Constant  Value=VonKarman.phi
  Cos1 : Trigonometry  Operator=cos
  Divide{1..6} (6 alike) : Product  Inputs=**
  Gain : Gain  Gain=VonKarman.alpha
  Gain1 : Gain  Gain=2*VonKarman.df
  Gain2 : Gain  Gain=2*pi
  Sqrt : Sqrt
  Square : Math  Operator=square
  Square1 : Math  Operator=square
  Step : Step  SampleTime=0
  Sv : Subsystem
  Transfer Fcn : TransferFcn  Numerator=[100]  Denominator=conv([1 10], [1 10])
  X : Subsystem
  d_out : Outport
  d_in : Outport  Port=2
  wires:
  Divide1/1 -> Transfer Fcn/1
  Cos1/1 -> Divide3/1
  Step/1 -> Divide1/2
  Divide4/1 -> Add2/1
  Gain1/1 -> Sqrt/1
  X/1(Out_X) -> Square/1
  Sqrt/1 -> Divide5/1
  Gain2/1 -> Divide4/2
  Clock2/1 -> Divide4/1
  Sv/1(Out_Sv) -> Divide2/2
  Constant2/1 -> Square1/1
  Add2/1 -> Cos1/1
  Divide2/1 -> Gain1/1
  Divide3/1 -> Add/1
  Square/1 -> Divide2/1
  Add/1 -> Divide1/1
  Constant1/1 -> Divide6/1
  Constant3/1 -> X/1(f), Sv/1(f), Gain2/1
  Divide5/1 -> Divide3/2
  Constant4/1 -> Add2/2
  Square1/1 -> Divide6/2
  Divide6/1 -> Divide5/2
  Transfer Fcn/1 -> Gain/1
  Constant/1 -> d_out/1
  Gain/1 -> d_in/1

== system Telescope_model_PID/Telescope Model/Elevation Model/Noise Model/White Noise Output ==
  Band-Limited White Noise : simulink/Sources/Band-Limited White Noise  Cov=[0.04]  Ts=0.02  seed=[23341]
  Band-Limited White Noise1 : simulink/Sources/Band-Limited White Noise  Cov=400000  Ts=0.02  seed=[23341]
  Constant1 : Constant  Value=0
  Gain : Gain  Gain=Deg2Arcs
  Scope : Scope  NumInputPorts=3
  d_out : Outport
  d_in : Outport  Port=2
  wires:
  Band-Limited White Noise/1 -> Scope/1, Gain/1
  Band-Limited White Noise1/1 -> Scope/2
  Gain/1 -> Scope/3, d_out/1
  Constant1/1 -> d_in/1

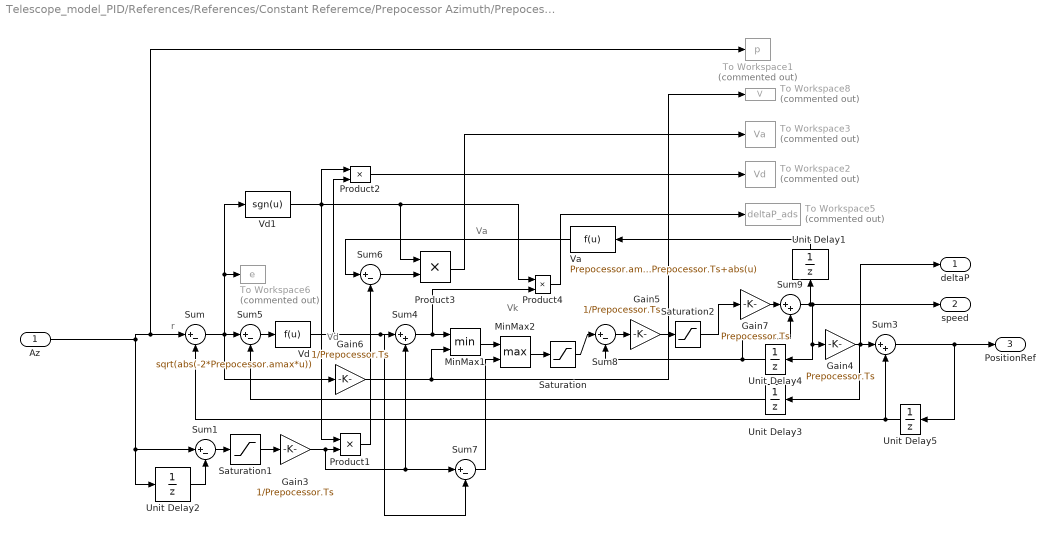
== system Telescope_model_PID/References/References/Constant Referemce/Prepocessor Azimuth/Prepocessor Elevation ==
  note: Vd
  note: Va
  note: Vk
  note: r
  Az : Inport
  Gain3 : Gain  Gain=1/Prepocessor.Ts
  Gain4 : Gain  Gain=Prepocessor.Ts
  Gain5 : Gain  Gain=1/Prepocessor.Ts
  Gain6 : Gain  Gain=1/Prepocessor.Ts
  Gain7 : Gain  Gain=Prepocessor.Ts
  MinMax1 : MinMax  Inputs=2
  MinMax2 : MinMax  Function=max  Inputs=2
  Product{1..4} (4 alike) : Product
  Saturation : Saturate  UpperLimit=Prepocessor.vmax  LowerLimit=-Prepocessor.vmax
  Saturation1 : Saturate  UpperLimit=Prepocessor.vmax*Prepocessor.Ts  LowerLimit=-Prepocessor.vmax*Prepocessor.Ts
  Saturation2 : Saturate  UpperLimit=Prepocessor.amax  LowerLimit=-Prepocessor.amax
  Sum{,1,5..8} (6 alike) : Sum  Inputs=|+-
  Sum3 : Sum  Inputs=|++
  Sum4 : Sum  Inputs=|++
  Sum9 : Sum  Inputs=|++
  To Workspace1 : ToWorkspace  Commented=on  VariableName=p  SampleTime=-1
  To Workspace2 : ToWorkspace  Commented=on  VariableName=Vd  SampleTime=-1
  To Workspace3 : ToWorkspace  Commented=on  VariableName=Va  SampleTime=-1
  To Workspace5 : ToWorkspace  Commented=on  VariableName=deltaP_ads  SampleTime=-1
  To Workspace6 : ToWorkspace  Commented=on  VariableName=e  SampleTime=-1
  To Workspace8 : ToWorkspace  Commented=on  VariableName=V  SampleTime=-1
  Unit Delay{1..4} (4 alike) : UnitDelay  SampleTime=-1  HasFrameUpgradeWarning=on
  Unit Delay5 : UnitDelay  InitialCondition=Prepocessor.p0az  SampleTime=-1  HasFrameUpgradeWarning=on
  Va : Fcn  Expr=Prepocessor.amax*Prepocessor.Ts+abs(u)
  Vd : Fcn  Expr=sqrt(abs(-2*Prepocessor.amax*u))
  Vd1 : Fcn  Expr=sgn(u)
  deltaP : Outport
  speed : Outport  Port=2
  PositionRef : Outport  Port=3
  wires:
  Unit Delay5/1 -> Sum/2, Sum3/2
  Product4/1 -> To Workspace5/1
  Az/1 -> Unit Delay2/1, Sum1/1, Sum/1, To Workspace1/1
  Product2/1 -> To Workspace2/1
  Product3/1 -> To Workspace3/1
  Vd/1 -> Product2/2, Sum7/2, Sum4/1
  Sum4/1 -> Product4/2, MinMax1/1
  Unit Delay3/1 -> Sum5/2
  Product1/1 -> Sum6/2
  Gain4/1 -> deltaP/1, Sum3/1, Unit Delay3/1
  Vd1/1 -> Product2/1, Product1/1, Product4/1, Product3/1
  Saturation2/1 -> Gain7/1
  Sum7/1 -> MinMax2/2
  Va/1 -> Sum6/1
  Sum1/1 -> Saturation1/1
  Sum/1 -> Sum5/1, Gain6/1, Vd1/1, To Workspace6/1
  Unit Delay2/1 -> Sum1/2
  Gain7/1 -> Sum9/1
  Sum9/1 -> speed/1, Unit Delay4/1, Gain4/1, Unit Delay1/1
  Unit Delay4/1 -> Sum8/2, Sum9/2
  Gain6/1 -> MinMax1/2, To Workspace8/1
  MinMax1/1 -> MinMax2/1
  Gain3/1 -> Sum7/1, Sum4/2, Product1/2
  Sum6/1 -> Product3/2
  Saturation1/1 -> Gain3/1
  Saturation/1 -> Sum8/1
  Sum8/1 -> Gain5/1
  Sum5/1 -> Vd/1
  MinMax2/1 -> Saturation/1
  Unit Delay1/1 -> Va/1
  Gain5/1 -> Saturation2/1
  Sum3/1 -> Unit Delay5/1, PositionRef/1

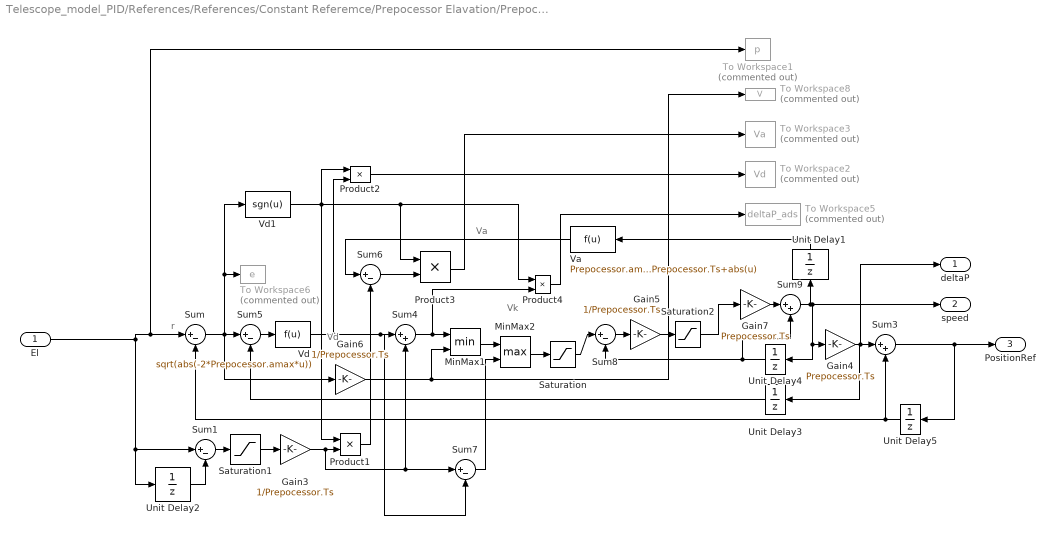
== system Telescope_model_PID/References/References/Constant Referemce/Prepocessor Elavation/Prepocessor Elevation ==
  note: Vd
  note: Va
  note: Vk
  note: r
  El : Inport
  Gain3 : Gain  Gain=1/Prepocessor.Ts
  Gain4 : Gain  Gain=Prepocessor.Ts
  Gain5 : Gain  Gain=1/Prepocessor.Ts
  Gain6 : Gain  Gain=1/Prepocessor.Ts
  Gain7 : Gain  Gain=Prepocessor.Ts
  MinMax1 : MinMax  Inputs=2
  MinMax2 : MinMax  Function=max  Inputs=2
  Product{1..4} (4 alike) : Product
  Saturation : Saturate  UpperLimit=Prepocessor.vmax  LowerLimit=-Prepocessor.vmax
  Saturation1 : Saturate  UpperLimit=Prepocessor.vmax*Prepocessor.Ts  LowerLimit=-Prepocessor.vmax*Prepocessor.Ts
  Saturation2 : Saturate  UpperLimit=Prepocessor.amax  LowerLimit=-Prepocessor.amax
  Sum{,1,5..8} (6 alike) : Sum  Inputs=|+-
  Sum3 : Sum  Inputs=|++
  Sum4 : Sum  Inputs=|++
  Sum9 : Sum  Inputs=|++
  To Workspace1 : ToWorkspace  Commented=on  VariableName=p  SampleTime=-1
  To Workspace2 : ToWorkspace  Commented=on  VariableName=Vd  SampleTime=-1
  To Workspace3 : ToWorkspace  Commented=on  VariableName=Va  SampleTime=-1
  To Workspace5 : ToWorkspace  Commented=on  VariableName=deltaP_ads  SampleTime=-1
  To Workspace6 : ToWorkspace  Commented=on  VariableName=e  SampleTime=-1
  To Workspace8 : ToWorkspace  Commented=on  VariableName=V  SampleTime=-1
  Unit Delay{1..4} (4 alike) : UnitDelay  SampleTime=-1  HasFrameUpgradeWarning=on
  Unit Delay5 : UnitDelay  InitialCondition=Prepocessor.p0el  SampleTime=-1  HasFrameUpgradeWarning=on
  Va : Fcn  Expr=Prepocessor.amax*Prepocessor.Ts+abs(u)
  Vd : Fcn  Expr=sqrt(abs(-2*Prepocessor.amax*u))
  Vd1 : Fcn  Expr=sgn(u)
  deltaP : Outport
  speed : Outport  Port=2
  PositionRef : Outport  Port=3
  wires:
  Unit Delay5/1 -> Sum/2, Sum3/2
  Product4/1 -> To Workspace5/1
  El/1 -> Unit Delay2/1, Sum1/1, Sum/1, To Workspace1/1
  Product2/1 -> To Workspace2/1
  Product3/1 -> To Workspace3/1
  Vd/1 -> Product2/2, Sum7/2, Sum4/1
  Sum4/1 -> Product4/2, MinMax1/1
  Unit Delay3/1 -> Sum5/2
  Product1/1 -> Sum6/2
  Gain4/1 -> deltaP/1, Sum3/1, Unit Delay3/1
  Vd1/1 -> Product2/1, Product1/1, Product4/1, Product3/1
  Saturation2/1 -> Gain7/1
  Sum7/1 -> MinMax2/2
  Va/1 -> Sum6/1
  Sum1/1 -> Saturation1/1
  Sum/1 -> Sum5/1, Gain6/1, Vd1/1, To Workspace6/1
  Unit Delay2/1 -> Sum1/2
  Gain7/1 -> Sum9/1
  Sum9/1 -> speed/1, Unit Delay4/1, Gain4/1, Unit Delay1/1
  Unit Delay4/1 -> Sum8/2, Sum9/2
  Gain6/1 -> MinMax1/2, To Workspace8/1
  MinMax1/1 -> MinMax2/1
  Gain3/1 -> Sum7/1, Sum4/2, Product1/2
  Sum6/1 -> Product3/2
  Saturation1/1 -> Gain3/1
  Saturation/1 -> Sum8/1
  Sum8/1 -> Gain5/1
  Sum5/1 -> Vd/1
  MinMax2/1 -> Saturation/1
  Unit Delay1/1 -> Va/1
  Gain5/1 -> Saturation2/1
  Sum3/1 -> Unit Delay5/1, PositionRef/1

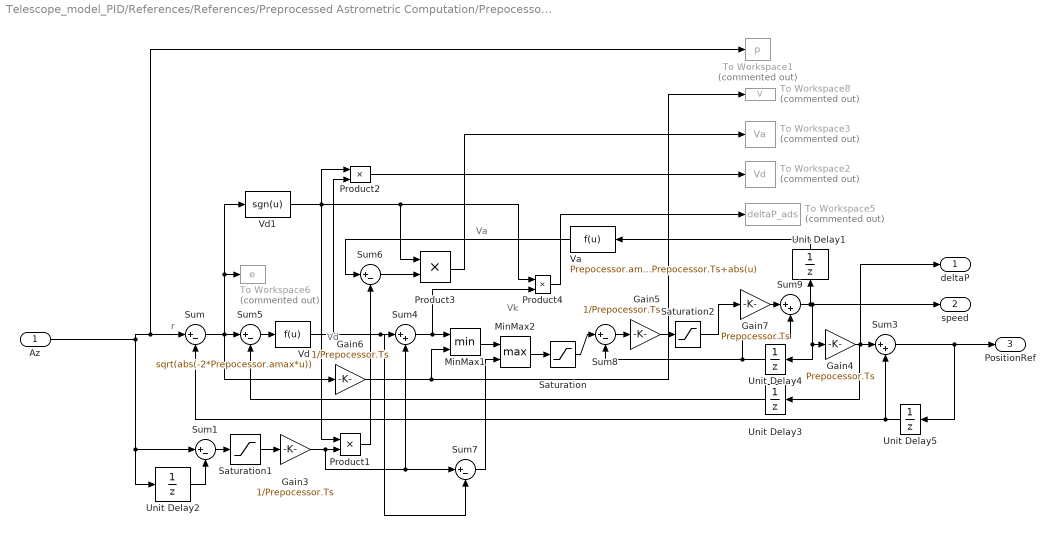
== system Telescope_model_PID/References/References/Preprocessed Astrometric Computation/Prepocessor Azimuth/Prepocessor Elevation ==
  note: Vd
  note: Va
  note: Vk
  note: r
  Az : Inport
  Gain3 : Gain  Gain=1/Prepocessor.Ts
  Gain4 : Gain  Gain=Prepocessor.Ts
  Gain5 : Gain  Gain=1/Prepocessor.Ts
  Gain6 : Gain  Gain=1/Prepocessor.Ts
  Gain7 : Gain  Gain=Prepocessor.Ts
  MinMax1 : MinMax  Inputs=2
  MinMax2 : MinMax  Function=max  Inputs=2
  Product{1..4} (4 alike) : Product
  Saturation : Saturate  UpperLimit=Prepocessor.vmax  LowerLimit=-Prepocessor.vmax
  Saturation1 : Saturate  UpperLimit=Prepocessor.vmax*Prepocessor.Ts  LowerLimit=-Prepocessor.vmax*Prepocessor.Ts
  Saturation2 : Saturate  UpperLimit=Prepocessor.amax  LowerLimit=-Prepocessor.amax
  Sum{,1,5..8} (6 alike) : Sum  Inputs=|+-
  Sum3 : Sum  Inputs=|++
  Sum4 : Sum  Inputs=|++
  Sum9 : Sum  Inputs=|++
  To Workspace1 : ToWorkspace  Commented=on  VariableName=p  SampleTime=-1
  To Workspace2 : ToWorkspace  Commented=on  VariableName=Vd  SampleTime=-1
  To Workspace3 : ToWorkspace  Commented=on  VariableName=Va  SampleTime=-1
  To Workspace5 : ToWorkspace  Commented=on  VariableName=deltaP_ads  SampleTime=-1
  To Workspace6 : ToWorkspace  Commented=on  VariableName=e  SampleTime=-1
  To Workspace8 : ToWorkspace  Commented=on  VariableName=V  SampleTime=-1
  Unit Delay{1..4} (4 alike) : UnitDelay  SampleTime=-1  HasFrameUpgradeWarning=on
  Unit Delay5 : UnitDelay  InitialCondition=Prepocessor.p0az  SampleTime=-1  HasFrameUpgradeWarning=on
  Va : Fcn  Expr=Prepocessor.amax*Prepocessor.Ts+abs(u)
  Vd : Fcn  Expr=sqrt(abs(-2*Prepocessor.amax*u))
  Vd1 : Fcn  Expr=sgn(u)
  deltaP : Outport
  speed : Outport  Port=2
  PositionRef : Outport  Port=3
  wires:
  Unit Delay5/1 -> Sum/2, Sum3/2
  Product4/1 -> To Workspace5/1
  Az/1 -> Unit Delay2/1, Sum1/1, Sum/1, To Workspace1/1
  Product2/1 -> To Workspace2/1
  Product3/1 -> To Workspace3/1
  Vd/1 -> Product2/2, Sum7/2, Sum4/1
  Sum4/1 -> Product4/2, MinMax1/1
  Unit Delay3/1 -> Sum5/2
  Product1/1 -> Sum6/2
  Gain4/1 -> deltaP/1, Sum3/1, Unit Delay3/1
  Vd1/1 -> Product2/1, Product1/1, Product4/1, Product3/1
  Saturation2/1 -> Gain7/1
  Sum7/1 -> MinMax2/2
  Va/1 -> Sum6/1
  Sum1/1 -> Saturation1/1
  Sum/1 -> Sum5/1, Gain6/1, Vd1/1, To Workspace6/1
  Unit Delay2/1 -> Sum1/2
  Gain7/1 -> Sum9/1
  Sum9/1 -> speed/1, Unit Delay4/1, Gain4/1, Unit Delay1/1
  Unit Delay4/1 -> Sum8/2, Sum9/2
  Gain6/1 -> MinMax1/2, To Workspace8/1
  MinMax1/1 -> MinMax2/1
  Gain3/1 -> Sum7/1, Sum4/2, Product1/2
  Sum6/1 -> Product3/2
  Saturation1/1 -> Gain3/1
  Saturation/1 -> Sum8/1
  Sum8/1 -> Gain5/1
  Sum5/1 -> Vd/1
  MinMax2/1 -> Saturation/1
  Unit Delay1/1 -> Va/1
  Gain5/1 -> Saturation2/1
  Sum3/1 -> Unit Delay5/1, PositionRef/1
